simulink model "Damping_Moment"  (R2023a)
settings: Solver=VariableStepAuto  StartTime=0.0  StopTime=10.0  RelTol=1e-3
values from neighbouring files (symbols this model uses):
  a = 340.3    [Roll_variables.mat]
  rho = 1.225    [Roll_variables.mat]
settings Model: Creator=kwood  LastModifiedBy=A-0001

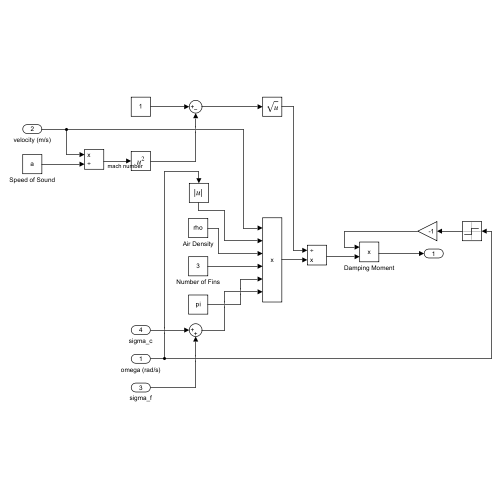
[thumbnail: Simulink's stored preview of the top-level diagram]
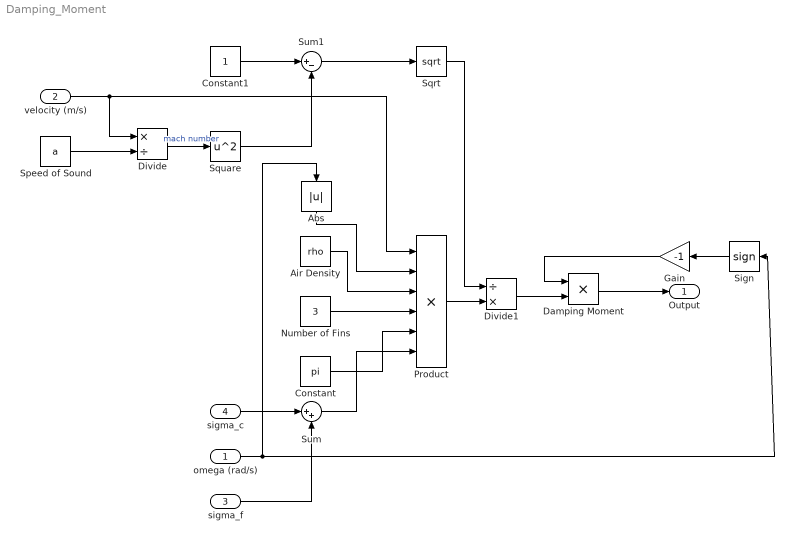
== system Damping_Moment ==
  omega (rad/s) : Inport
  velocity (m/s) : Inport  Port=2
  sigma_f : Inport  Port=3
  sigma_c : Inport  Port=4
  Abs : Abs  SaturateOnIntegerOverflow=off
  Air Density : Constant  Value=rho
  Constant : Constant  Value=pi
  Constant1 : Constant
  Damping Moment : Product
  Divide : Product  Inputs=*/
  Divide1 : Product  Inputs=/*
  Gain : Gain  Gain=-1
  Number of Fins : Constant  Value=3
  Product : Product  Inputs=6
  Sign : Signum
  Speed of Sound : Constant  Value=a
  Sqrt : Sqrt
  Square : Math  Operator=square
  Sum : Sum  Inputs=|++
  Sum1 : Sum  Inputs=|+-
  Output : Outport
  wires:
  velocity (m/s)/1 -> Product/1, Divide/1
  sigma_f/1 -> Sum/2
  Speed of Sound/1 -> Divide/2
  Divide/1 -> Square/1  "mach number"
  Constant1/1 -> Sum1/1
  omega (rad/s)/1 -> Abs/1, Sign/1
  Square/1 -> Sum1/2
  sigma_c/1 -> Sum/1
  Abs/1 -> Product/2
  Sum1/1 -> Sqrt/1
  Air Density/1 -> Product/3
  Number of Fins/1 -> Product/4
  Constant/1 -> Product/5
  Sum/1 -> Product/6
  Sqrt/1 -> Divide1/1
  Product/1 -> Divide1/2
  Divide1/1 -> Damping Moment/2
  Damping Moment/1 -> Output/1
  Gain/1 -> Damping Moment/1
  Sign/1 -> Gain/1
